simulink model "stepcomp"  (R2019b)
settings: Solver=VariableStepAuto  StartTime=0.0  StopTime=10.0  RelTol=1e-3
libraries: simulink_extras x3
settings Model: Creator=muafi  LastModifiedBy=muafi

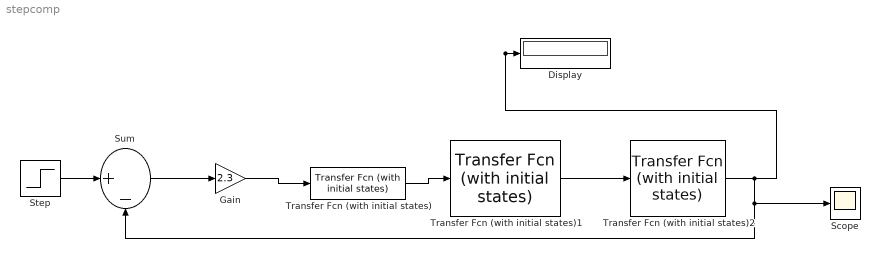
== system stepcomp ==
  Display : Display
      settings: Format=decimal (Stored Integer)  Decimation=2
  Gain : Gain  Gain=2.3
  Scope : Scope
  Step : Step  Time=10  Before=3  After=0  SampleTime=0
  Sum : Sum  Inputs=|+-
  Transfer Fcn (with initial states) : simulink_extras/Additional Linear/Transfer Fcn (with initial states)  N=[13.3 30.058]  D=[1 30]  X0=0
  Transfer Fcn (with initial states)1 : simulink_extras/Additional Linear/Transfer Fcn (with initial states)  N=[-2750]  D=[1 42.3 2750]  X0=0
  Transfer Fcn (with initial states)2 : simulink_extras/Additional Linear/Transfer Fcn (with initial states)  N=[-7.21]  D=[1 0.12 -2.368]  X0=0
  wires:
  Step/1 -> Sum/1
  Sum/1 -> Gain/1
  Gain/1 -> Transfer Fcn (with initial states)/1
  Transfer Fcn (with initial states)/1 -> Transfer Fcn (with initial states)1/1
  Transfer Fcn (with initial states)1/1 -> Transfer Fcn (with initial states)2/1
  Transfer Fcn (with initial states)2/1 -> Display/1, Sum/2, Scope/1
